simulink model "simulation_diego_perea"  (R2020a)
settings: Solver=VariableStepAuto  StartTime=0.0  StopTime=5  RelTol=1e-3
values from neighbouring files (symbols this model uses):
  a = eval(aj)    [Proyecto_diego_perea_control2.m]
  b = [1/10;0;0]    [Proyecto_diego_perea_control2.m]
  c = [0,0,1]    [Proyecto_diego_perea_control2.m]
  d = 0    [Proyecto_diego_perea_control2.m]
  h = h'    [Proyecto_diego_perea_control2.m]
  hdis = hdis'    [Proyecto_diego_perea_control2.m]
  k = place(a,b,pd)    [Proyecto_diego_perea_control2.m]
  kdis = place(adis,bdis,polosdiscredes)    [Proyecto_diego_perea_control2.m]
  ki = kt(1:1,4:4)    [Proyecto_diego_perea_control2.m]
  kidis = ktdis(:,4:4)    [Proyecto_diego_perea_control2.m]
  kp = kt(1:1,1:3)    [Proyecto_diego_perea_control2.m]
  kpdis = ktdis(:,1:3)    [Proyecto_diego_perea_control2.m]
  tm = 0.1    [Proyecto_diego_perea_control2.m]
undefined symbols (not defined in the file or in its folder): adis, bdis, cdis
settings Model: Creator=estra  LastModifiedBy=User

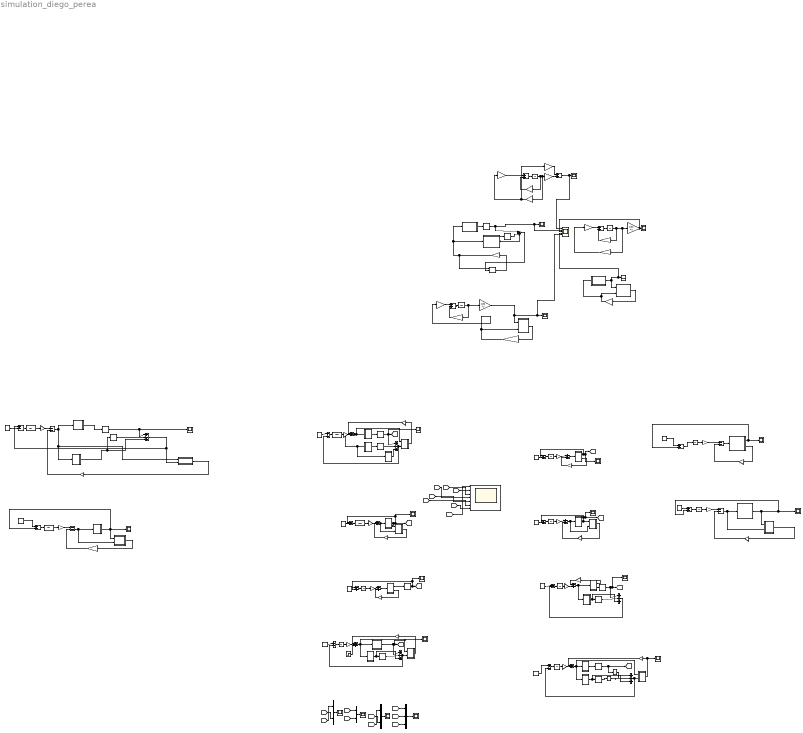
== system simulation_diego_perea ==
  note: TRACKERS (DISCRETE , CONTINUOS -SMITH)
  note: DIEGO IVAN PEREA MONTEALEGRE
  note: Continuous plant Regulator
  note: Continuous plant with regulator discrete
  note: REGULATORS
  note: Continuous plant regulator with observer
  note: Regulator with continuous plant ,observe and predictor smith.
  note: Discrete regulator with non_linear plant and with observer in discrete
  note: Tracker in discrete with linear plant and with observer in discrete
  note: Tracker with linear plant
  note: Tracker with linear plant and observer
  note: Tracker in discrete with linear plant in discrete with observer in discrete
  note: Tracker with linear plant and observer
  note: Tracker with linear plant
  note: Tracker in discrete with linear plant in discrete with observer in discrete
  note: Tracker in discrete with linear plant and with observer in discrete
  note: Plant with retard
  note: Tracker with retard smith
  note: Tracker observer smith
  note: Tracker observer smith with external perturbation
  -kp{,1,4..5,7,9} (6 alike) : Gain  Gain=-kp  Multiplication=Matrix(K*u) (u vector)
  -kp3 : Gain  Gain=-kpdis  Multiplication=Matrix(K*u) (u vector)  SampleTime=tm
  -kp6 : Gain  Gain=-kpdis  Multiplication=Matrix(K*u) (u vector)  SampleTime=tm
  Add : Sum
  Add{1,8,24,44} (4 alike) : Sum  Inputs=+-
  Add14 : Sum
  Add{6,9,25,45} (4 alike) : Sum  Inputs=--
  Add7 : Sum
  Constant{,1,3..4,6..7,9..11,21} (10 alike) : Constant
  Constant5 : Constant  SampleTime=tm
  Constant8 : Constant  SampleTime=tm
  "Continuous plant Regulator " : Sum
  Continuous plant regulator with observer : Subsystem
  "Continuous plant with regulator  discrete " : Gain  Gain=cdis  Multiplication=Matrix(K*u) (u vector)
  Discrete Transfer Fcn1 : DiscreteTransferFcn  Numerator=[1 0]  Denominator=[1 -1]  SampleTime=tm
  Discrete Transfer Fcn10 : DiscreteTransferFcn  Numerator=[1,0]  Denominator=[1 -1]  SampleTime=tm
  Discrete Transfer Fcn3 : DiscreteTransferFcn  Numerator=[1 0]  Denominator=[1 -1]  SampleTime=tm
  Discrete Transfer Fcn6 : DiscreteTransferFcn  Numerator=[1,0]  Denominator=[1 -1]  SampleTime=tm
  Discrete regulator with non_linear plant and with observer in discrete : Gain  Gain=cdis  Multiplication=Matrix(K*u) (u vector)
  Gain{,1,5..6,8,10} (6 alike) : Gain  Gain=-ki  Multiplication=Matrix(K*u) (u vector)
  Gain4 : Gain  Gain=-kidis  Multiplication=Matrix(K*u) (u vector)  SampleTime=tm
  Gain7 : Gain  Gain=-kidis  Multiplication=Matrix(K*u) (u vector)  SampleTime=tm
  Integrator : Integrator  InitialCondition=5
  Integrator{1..8} (8 alike) : Integrator
  Mux : Mux  Inputs=2
  Mux1 : Mux  Inputs=2
  Mux2 : Mux  Inputs=2
  Mux3 : Mux  Inputs=3
  Ob_predictor_smith_regulator : Subsystem
  Observer_1 : Subsystem
  Plant  with retard : TransportDelay
  Planta lineal continua12 : Subsystem
  Planta lineal continua2 : Subsystem
  Planta lineal continua3 : Subsystem
  Planta lineal continua4 : Subsystem
  Planta lineal continua7 : Subsystem
  Planta lineal continua8 : Subsystem
  Planta lineal discreta3 : Subsystem
  Planta lineal discreta4 : Subsystem
  Planta lineal discreta5 : Subsystem
  Regulator_continuos_observe_preditor smith : TransportDelay
  Retardo de la planta{1,3,5,7} (4 alike) : TransportDelay
  Scope : Scope  NumInputPorts=7
  Scope{1..10,12..22} (21 alike) : Scope
  Scope11 : Scope  NumInputPorts=5
  Step : Step  Time=0  After=0  SampleTime=0
  Sum{,7,15..16,21,26} (6 alike) : Sum  Inputs=|+-+
  Sum{1,3,8,17} (4 alike) : Sum  Inputs=|-+
  Sum{10,12,14,24} (4 alike) : Sum  Inputs=|+-
  Sum{2,4,9,11,13,18..19} (7 alike) : Sum  Inputs=|++
  Sum25 : Sum  Inputs=|+++
  Tracker  observer smith with external  perturbation : Subsystem
  Tracker  with retard smith : TransportDelay
  Tracker in discrete with linear plant and with observer in discrete : TransportDelay
  Tracker in discrete with linear plant and with observer in discrete1 : TransportDelay  DelayTime=0.8
  Tracker in discrete with linear plant in discrete with observer in discrete : Subsystem
  Tracker in discrete with linear plant in discrete with observer in discrete1 : Subsystem
  Tracker observer smith : TransportDelay
  Tracker with linear plant : Subsystem
  Tracker with linear plant and observer : Subsystem
  Tracker with linear plant and observer1 : Subsystem
  Tracker with linear plant1 : Subsystem
  Transfer Fcn : TransferFcn  Denominator=[50 1]
  Transfer Fcn1 : TransferFcn  Denominator=[50,1]
  Transport Delay1 : TransportDelay
  Transport Delay15 : TransportDelay  DelayTime=0.8
  Unit Delay : UnitDelay  InitialCondition=-8  SampleTime=tm  HasFrameUpgradeWarning=on
  Unit Delay1 : UnitDelay  InitialCondition=-8  SampleTime=tm  HasFrameUpgradeWarning=on
  a : Gain  Gain=a  Multiplication=Matrix(K*u) (u vector)
  adis : Gain  Gain=adis  Multiplication=Matrix(K*u) (u vector)
  adis1 : Gain  Gain=adis  Multiplication=Matrix(K*u) (u vector)
  b : Gain  Gain=b  Multiplication=Matrix(K*u) (u vector)
  bdis : Gain  Gain=bdis  Multiplication=Matrix(K*u) (u vector)
  bdis1 : Gain  Gain=bdis  Multiplication=Matrix(K*u) (u vector)
  c : Gain  Gain=c  Multiplication=Matrix(K*u) (u vector)
  continuous plant 6 : Subsystem
  continuous plant _ j : Subsystem
  d : Gain  Gain=d  Multiplication=Matrix(K*u) (u vector)
  k : Gain  Gain=-k  Multiplication=Matrix(K*u) (u vector)
  k3 : Gain  Gain=-k  Multiplication=Matrix(K*u) (u vector)
  k6 : Gain  Gain=-kdis  Multiplication=Matrix(K*u) (u vector)
  k8 : Gain  Gain=-k  Multiplication=Matrix(K*u) (u vector)
  kdis : Gain  Gain=-kdis  Multiplication=Matrix(K*u) (u vector)
  ki2 : Gain  Gain=ki  Multiplication=Matrix(K*u) (u vector)
  ki3 : Gain  Gain=ki  Multiplication=Matrix(K*u) (u vector)
  kidis10 : Gain  Gain=kidis  Multiplication=Matrix(K*u) (u vector)
  kidis6 : Gain  Gain=kidis  Multiplication=Matrix(K*u) (u vector)
  kp3 : Gain  Gain=kp  Multiplication=Matrix(K*u) (u vector)
  kp4 : Gain  Gain=kp  Multiplication=Matrix(K*u) (u vector)
  kpdis3 : Gain  Gain=kpdis  Multiplication=Matrix(K*u) (u vector)
  kpdis7 : Gain  Gain=kpdis  Multiplication=Matrix(K*u) (u vector)
  ob_discr_11 : Subsystem
  observador1 : Subsystem
  observador2 : Subsystem
  observador3 : Subsystem
  observadordis : Subsystem
  observadordis2 : Subsystem
  observer10 : Subsystem
  observer18 : Subsystem
  observer3 : Subsystem
  plant_1 : Subsystem
  planta13 : Subsystem
  wires:
  Continuous plant regulator with observer/1(Out1) -> Scope11/4, Scope10/1, Observer_1/1(In2)
  k3/1 -> Continuous plant regulator with observer/1(In1), Observer_1/2(In1)
  Observer_1/1(Out1) -> k3/1
  Transport Delay1/1 -> Sum/2
  plant_1/1(Out1) -> Transport Delay1/1, Sum/3
  k8/1 -> continuous plant _ j/1(In1), plant_1/1(In1), Ob_predictor_smith_regulator/1(In1)
  Ob_predictor_smith_regulator/1(Out1) -> k8/1
  Regulator_continuos_observe_preditor smith/1 -> Scope11/2, Scope8/1, Sum/1
  continuous plant _ j/1(Out1) -> Regulator_continuos_observe_preditor smith/1
  Sum/1 -> Ob_predictor_smith_regulator/2(In2)
  c/1 -> "Continuous plant Regulator "/2
  Add/1 -> Integrator/1
  b/1 -> Add/1
  a/1 -> Add/2
  k/1 -> d/1, b/1
  d/1 -> "Continuous plant Regulator "/1
  Integrator/1 -> a/1, k/1, c/1
  kdis/1 -> bdis/1
  adis/1 -> Add14/2
  Add14/1 -> Unit Delay/1
  Unit Delay/1 -> kdis/1, "Continuous plant with regulator  discrete "/1, adis/1
  bdis/1 -> Add14/1
  k6/1 -> bdis1/1, ob_discr_11/2(In1)
  ob_discr_11/1(Out1) -> k6/1
  continuous plant 6/1(Out1) -> Tracker in discrete with linear plant and with observer in discrete1/1
  Constant21/1 -> Add44/1
  Sum7/1 -> observer18/2(In2), Add44/2
  kidis10/1 -> Add45/1
  observer18/1(Out1) -> kpdis7/1
  Tracker in discrete with linear plant and with observer in discrete1/1 -> Scope3/1, Sum7/1
  Add44/1 -> Discrete Transfer Fcn10/1
  Discrete Transfer Fcn10/1 -> kidis10/1
  Add45/1 -> planta13/1(In1), observer18/1(In1), continuous plant 6/1(In1)
  kpdis7/1 -> Add45/2
  Transport Delay15/1 -> Sum7/2
  planta13/1(Out1) -> Sum7/3, Transport Delay15/1
  Add6/1 -> Tracker with linear plant1/1(In1)
  kp4/1 -> Add6/2
  Tracker with linear plant1/2(Output) -> kp4/1
  Integrator1/1 -> ki3/1
  Add1/1 -> Integrator1/1
  ki3/1 -> Add6/1
  Constant3/1 -> Add1/1
  Add9/1 -> observer3/2(In1), Tracker with linear plant and observer1/1(In1)
  kp3/1 -> Add9/2
  Constant4/1 -> Add8/1
  observer3/1(Out1) -> kp3/1
  Integrator7/1 -> ki2/1
  Add8/1 -> Integrator7/1
  ki2/1 -> Add9/1
  Tracker with linear plant and observer1/1(Out1) -> Scope12/1, Add8/2, observer3/1(In2)
  Tracker in discrete with linear plant in discrete with observer in discrete1/1(Out1) -> Scope4/1, observer10/1(In2), Add24/2
  kpdis3/1 -> Add25/2
  Add25/1 -> observer10/2(In1), Tracker in discrete with linear plant in discrete with observer in discrete1/1(In1)
  observer10/1(Out1) -> kpdis3/1
  Discrete Transfer Fcn6/1 -> kidis6/1
  Constant11/1 -> Add24/1
  kidis6/1 -> Add25/1
  Add24/1 -> Discrete Transfer Fcn6/1
  Discrete regulator with non_linear plant and with observer in discrete/1 -> Scope11/5, Scope9/1, ob_discr_11/1(In2)
  Tracker with linear plant1/1(Out1) -> Scope14/1, Add1/2
  Add7/1 -> Unit Delay1/1
  adis1/1 -> Add7/2
  Unit Delay1/1 -> Discrete regulator with non_linear plant and with observer in discrete/1, adis1/1
  bdis1/1 -> Add7/1
  "Continuous plant with regulator  discrete "/1 -> Scope11/3, Scope7/1
  "Continuous plant Regulator "/1 -> Scope11/1, Scope6/1
  Discrete Transfer Fcn3/1 -> Gain7/1
  Retardo de la planta7/1 -> Sum26/2
  -kp1/1 -> Sum4/2
  Planta lineal continua12/1(y) -> Sum26/3, Retardo de la planta7/1
  Sum25/1 -> Tracker  observer smith with external  perturbation/1(In1), observador3/1(u), Planta lineal continua12/1(u)
  Constant10/1 -> Sum24/1
  Constant8/1 -> Sum12/1
  Retardo de la planta1/1 -> Sum15/2
  Sum19/1 -> Planta lineal continua8/1(u), Planta lineal continua7/1(u)
  Planta lineal discreta5/1(y) -> Sum15/3
  Planta lineal continua8/1(y) -> Sum21/3, Retardo de la planta3/1
  Integrator4/1 -> Gain5/1
  Constant9/1 -> Sum14/1
  Tracker with linear plant/2(x) -> -kp/1
  Sum14/1 -> Integrator6/1
  Sum9/1 -> Tracker in discrete with linear plant in discrete with observer in discrete/1(u), observadordis/2(u)
  Gain4/1 -> Sum9/1
  Gain5/1 -> Sum18/1
  Sum18/1 -> Planta lineal continua2/1(u)
  Gain1/1 -> Sum4/1
  Sum8/1 -> Discrete Transfer Fcn1/1
  Integrator2/1 -> Gain/1
  Tracker  with retard smith/1 -> Sum21/1, Scope17/1, [A2]
  Integrator6/1 -> Gain8/1
  Planta lineal continua4/1(y) -> Sum16/3, Retardo de la planta5/1
  Planta lineal discreta4/1(y) -> Retardo de la planta1/1
  Retardo de la planta3/1 -> Sum21/2
  Sum1/1 -> Integrator2/1
  -kp4/1 -> Sum18/2
  [B1] -> Mux3/1
  -kp5/1 -> Sum11/1
  [C2] -> Mux3/2
  observadordis2/1(xgorro) -> -kp6/1
  Discrete Transfer Fcn1/1 -> Gain4/1
  -kp7/1 -> Sum19/1
  Constant5/1 -> Sum8/2
  Sum26/1 -> Sum24/2, observador3/2(y)
  [A1] -> Mux/2
  Sum11/1 -> Planta lineal continua4/1(u), Planta lineal continua3/1(u), observador2/1(u)
  Integrator3/1 -> Gain1/1
  Plant  with retard/1 -> Scope16/1, Sum17/1, [A1]
  Planta lineal continua7/1(x) -> -kp7/1
  [C1] -> Mux2/2
  -kp9/1 -> Sum25/1
  Sum12/1 -> Discrete Transfer Fcn3/1
  Gain10/1 -> Sum25/2
  [B1] -> Mux1/2
  Mux1/1 -> Scope13/1
  Sum24/1 -> Integrator8/1
  Mux/1 -> Scope5/1
  observador1/1(xgorro) -> -kp1/1
  Planta lineal discreta3/1(y) -> Tracker in discrete with linear plant and with observer in discrete/1
  Integrator8/1 -> Gain10/1
  Planta lineal continua2/1(y) -> Plant  with retard/1
  Sum15/1 -> Sum12/2, observadordis2/2(y)
  Sum3/1 -> Integrator3/1
  Integrator5/1 -> Gain6/1
  -kp3/1 -> Sum9/2
  Sum10/1 -> Integrator5/1
  Gain7/1 -> Sum13/2
  Planta lineal continua2/2(x) -> -kp4/1
  -kp/1 -> Sum2/2
  Tracker observer smith/1 -> Transfer Fcn1/1, [F]
  Tracker in discrete with linear plant and with observer in discrete/1 -> Scope21/1, Sum15/1, [C2]
  Retardo de la planta5/1 -> Transfer Fcn/1
  observadordis/1(xgorro) -> -kp3/1
  Constant1/1 -> Sum3/2
  Sum4/1 -> Tracker with linear plant and observer/1(u), observador1/2(u)
  Constant7/1 -> Sum10/1
  Mux3/1 -> Scope2/1
  [F] -> Mux3/3
  Step/1 -> Sum25/3
  Sum13/1 -> Planta lineal discreta3/1(u), observadordis2/1(u), Planta lineal discreta5/1(u), Planta lineal discreta4/1(u)
  observador3/1(xgorro) -> -kp9/1
  Tracker with linear plant/1(y) -> Sum1/1, [D], Scope15/1
  -kp6/1 -> Sum13/1
  Gain6/1 -> Sum11/2
  observador2/1(xgorro) -> Scope20/1, -kp5/1
  Sum17/1 -> Integrator4/1
  Sum16/1 -> observador2/2(y), Sum10/2
  Transfer Fcn1/1 -> Sum16/1
  Sum21/1 -> Sum14/2
  Gain8/1 -> Sum19/2
  Transfer Fcn/1 -> Sum16/2
  Constant/1 -> Sum1/2
  Constant6/1 -> Sum17/2
  Mux2/1 -> Scope1/1
  Tracker  observer smith with external  perturbation/1(Out1) -> Scope18/1, [B1], Sum26/1
  Sum2/1 -> Tracker with linear plant/1(u)
  [B] -> Mux1/1
  Planta lineal continua7/2(y) -> Tracker  with retard smith/1
  Planta lineal continua3/1(y) -> Tracker observer smith/1
  Gain/1 -> Sum2/1
  [A2] -> Mux/1
  [C2] -> Mux2/1
  Tracker in discrete with linear plant in discrete with observer in discrete/1(y) -> Scope19/1, Sum8/1, [C1], observadordis/1(y)
  Tracker with linear plant and observer/1(y) -> Scope22/1, [B], Sum3/1, observador1/1(y)
  [A2] -> Scope/2
  [B] -> Scope/3
  [B1] -> Scope/4
  [C1] -> Scope/5
  [C2] -> Scope/6
  [F] -> Scope/7
  [D] -> Scope/1

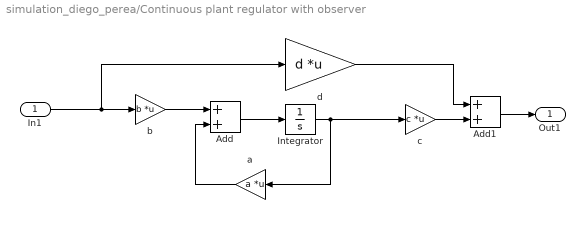
== system simulation_diego_perea/Continuous plant regulator with observer ==
  In1 : Inport
  Add : Sum
  Add1 : Sum
  Integrator : Integrator  InitialCondition=20
  a : Gain  Gain=a  Multiplication=Matrix(K*u) (u vector)
  b : Gain  Gain=b  Multiplication=Matrix(K*u) (u vector)
  c : Gain  Gain=c  Multiplication=Matrix(K*u) (u vector)
  d : Gain  Gain=d  Multiplication=Matrix(K*u) (u vector)
  Out1 : Outport
  wires:
  Integrator/1 -> c/1, a/1
  a/1 -> Add/2
  b/1 -> Add/1
  Add/1 -> Integrator/1
  In1/1 -> d/1, b/1
  c/1 -> Add1/2
  d/1 -> Add1/1
  Add1/1 -> Out1/1

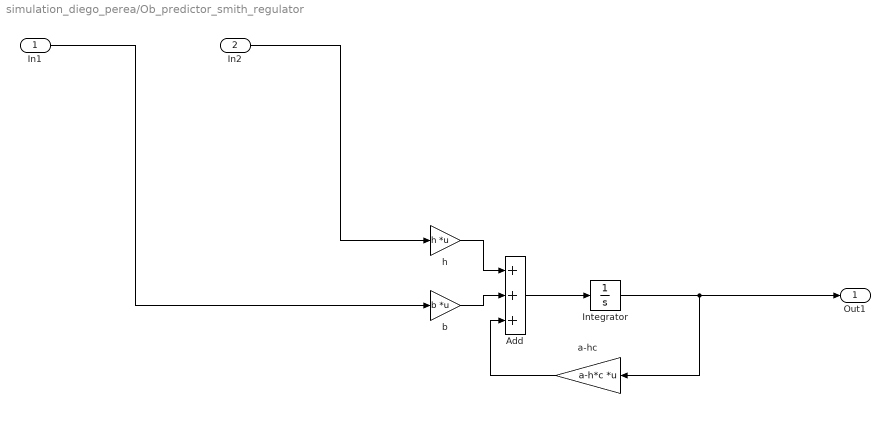
== system simulation_diego_perea/Ob_predictor_smith_regulator ==
  In1 : Inport
  In2 : Inport  Port=2
  Add : Sum  Inputs=+++
  Integrator : Integrator  InitialCondition=4
  a-hc : Gain  Gain=a-h*c  Multiplication=Matrix(K*u) (u vector)
  b : Gain  Gain=b  Multiplication=Matrix(K*u) (u vector)
  h : Gain  Gain=h  Multiplication=Matrix(K*u) (u vector)
  Out1 : Outport
  wires:
  a-hc/1 -> Add/3
  b/1 -> Add/2
  In2/1 -> h/1
  Integrator/1 -> Out1/1, a-hc/1
  In1/1 -> b/1
  Add/1 -> Integrator/1
  h/1 -> Add/1

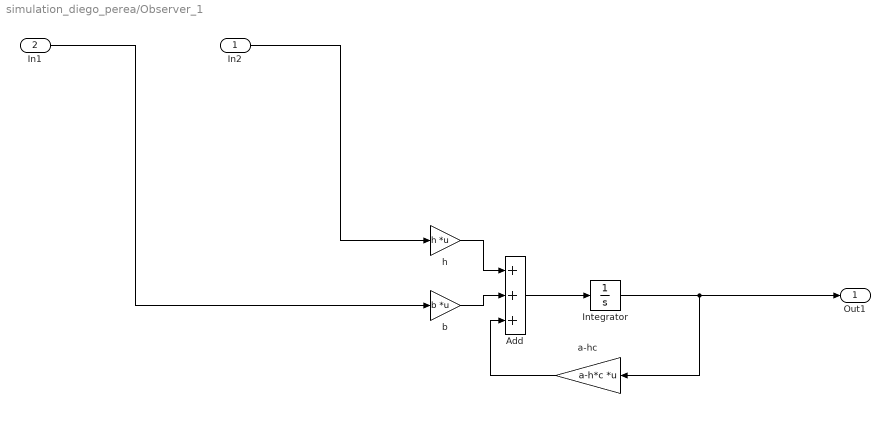
== system simulation_diego_perea/Observer_1 ==
  In2 : Inport
  In1 : Inport  Port=2
  Add : Sum  Inputs=+++
  Integrator : Integrator  InitialCondition=8
  a-hc : Gain  Gain=a-h*c  Multiplication=Matrix(K*u) (u vector)
  b : Gain  Gain=b  Multiplication=Matrix(K*u) (u vector)
  h : Gain  Gain=h  Multiplication=Matrix(K*u) (u vector)
  Out1 : Outport
  wires:
  a-hc/1 -> Add/3
  b/1 -> Add/2
  In2/1 -> h/1
  Integrator/1 -> Out1/1, a-hc/1
  In1/1 -> b/1
  Add/1 -> Integrator/1
  h/1 -> Add/1

== system simulation_diego_perea/Planta lineal continua12 ==
  u : Inport
  A : Gain  Gain=a  Multiplication=Matrix(K*u) (u vector)
  B : Gain  Gain=b  Multiplication=Matrix(K*u) (u vector)
  C : Gain  Gain=c  Multiplication=Matrix(K*u) (u vector)
  Integrator : Integrator
  Sum : Sum  Inputs=|++
  y : Outport
  wires:
  C/1 -> y/1
  u/1 -> B/1
  Integrator/1 -> C/1, A/1
  A/1 -> Sum/2
  Sum/1 -> Integrator/1
  B/1 -> Sum/1

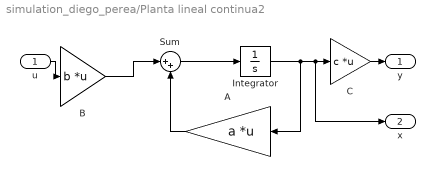
== system simulation_diego_perea/Planta lineal continua2 ==
  u : Inport
  A : Gain  Gain=a  Multiplication=Matrix(K*u) (u vector)
  B : Gain  Gain=b  Multiplication=Matrix(K*u) (u vector)
  C : Gain  Gain=c  Multiplication=Matrix(K*u) (u vector)
  Integrator : Integrator
  Sum : Sum  Inputs=|++
  y : Outport
  x : Outport  Port=2
  wires:
  C/1 -> y/1
  u/1 -> B/1
  Integrator/1 -> x/1, C/1, A/1
  A/1 -> Sum/2
  Sum/1 -> Integrator/1
  B/1 -> Sum/1

== system simulation_diego_perea/Planta lineal continua3 ==
  u : Inport
  A : Gain  Gain=a  Multiplication=Matrix(K*u) (u vector)
  B : Gain  Gain=b  Multiplication=Matrix(K*u) (u vector)
  C : Gain  Gain=c  Multiplication=Matrix(K*u) (u vector)
  Integrator : Integrator
  Sum : Sum  Inputs=|++
  y : Outport
  wires:
  B/1 -> Sum/1
  Sum/1 -> Integrator/1
  A/1 -> Sum/2
  Integrator/1 -> C/1, A/1
  u/1 -> B/1
  C/1 -> y/1

== system simulation_diego_perea/Planta lineal continua4 ==
  u : Inport
  A : Gain  Gain=a  Multiplication=Matrix(K*u) (u vector)
  B : Gain  Gain=b  Multiplication=Matrix(K*u) (u vector)
  C : Gain  Gain=c  Multiplication=Matrix(K*u) (u vector)
  Integrator : Integrator
  Sum : Sum  Inputs=|++
  y : Outport
  wires:
  B/1 -> Sum/1
  Sum/1 -> Integrator/1
  A/1 -> Sum/2
  Integrator/1 -> A/1, C/1
  u/1 -> B/1
  C/1 -> y/1

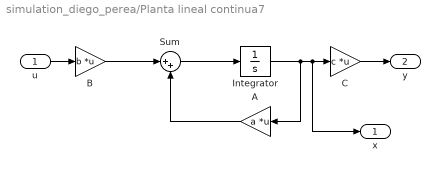
== system simulation_diego_perea/Planta lineal continua7 ==
  u : Inport
  A : Gain  Gain=a  Multiplication=Matrix(K*u) (u vector)
  B : Gain  Gain=b  Multiplication=Matrix(K*u) (u vector)
  C : Gain  Gain=c  Multiplication=Matrix(K*u) (u vector)
  Integrator : Integrator
  Sum : Sum  Inputs=|++
  x : Outport
  y : Outport  Port=2
  wires:
  u/1 -> B/1
  Integrator/1 -> x/1, C/1, A/1
  A/1 -> Sum/2
  Sum/1 -> Integrator/1
  B/1 -> Sum/1
  C/1 -> y/1

== system simulation_diego_perea/Planta lineal continua8 ==
  u : Inport
  A : Gain  Gain=a  Multiplication=Matrix(K*u) (u vector)
  B : Gain  Gain=b  Multiplication=Matrix(K*u) (u vector)
  C : Gain  Gain=c  Multiplication=Matrix(K*u) (u vector)
  Integrator : Integrator
  Sum : Sum  Inputs=|++
  y : Outport
  wires:
  B/1 -> Sum/1
  Sum/1 -> Integrator/1
  A/1 -> Sum/2
  Integrator/1 -> A/1, C/1
  u/1 -> B/1
  C/1 -> y/1

== system simulation_diego_perea/Planta lineal discreta3 ==
  u : Inport
  Sum4 : Sum  Inputs=|++
  Unit Delay : UnitDelay  SampleTime=-1  HasFrameUpgradeWarning=on
  adis : Gain  Gain=adis  Multiplication=Matrix(K*u) (u vector)  SampleTime=tm
  bdis : Gain  Gain=bdis  Multiplication=Matrix(K*u) (u vector)  SampleTime=tm
  cdis : Gain  Gain=cdis  Multiplication=Matrix(K*u) (u vector)  SampleTime=tm
  y : Outport
  wires:
  cdis/1 -> y/1
  u/1 -> bdis/1
  adis/1 -> Sum4/2
  Unit Delay/1 -> cdis/1, adis/1
  Sum4/1 -> Unit Delay/1
  bdis/1 -> Sum4/1

== system simulation_diego_perea/Planta lineal discreta4 ==
  u : Inport
  Sum4 : Sum  Inputs=|++
  Unit Delay : UnitDelay  SampleTime=-1  HasFrameUpgradeWarning=on
  adis : Gain  Gain=adis  Multiplication=Matrix(K*u) (u vector)  SampleTime=tm
  bdis : Gain  Gain=bdis  Multiplication=Matrix(K*u) (u vector)  SampleTime=tm
  cdis : Gain  Gain=cdis  Multiplication=Matrix(K*u) (u vector)  SampleTime=tm
  y : Outport
  wires:
  cdis/1 -> y/1
  u/1 -> bdis/1
  adis/1 -> Sum4/2
  Unit Delay/1 -> cdis/1, adis/1
  Sum4/1 -> Unit Delay/1
  bdis/1 -> Sum4/1

== system simulation_diego_perea/Planta lineal discreta5 ==
  u : Inport
  Sum4 : Sum  Inputs=|++
  Unit Delay : UnitDelay  SampleTime=-1  HasFrameUpgradeWarning=on
  adis : Gain  Gain=adis  Multiplication=Matrix(K*u) (u vector)  SampleTime=tm
  bdis : Gain  Gain=bdis  Multiplication=Matrix(K*u) (u vector)  SampleTime=tm
  cdis : Gain  Gain=cdis  Multiplication=Matrix(K*u) (u vector)  SampleTime=tm
  y : Outport
  wires:
  bdis/1 -> Sum4/1
  Sum4/1 -> Unit Delay/1
  Unit Delay/1 -> adis/1, cdis/1
  adis/1 -> Sum4/2
  u/1 -> bdis/1
  cdis/1 -> y/1

== system simulation_diego_perea/Tracker  observer smith with external  perturbation ==
  In1 : Inport
  Planta lineal continua11 : Subsystem
  Retardo de la planta8 : TransportDelay
  Out1 : Outport
  wires:
  Retardo de la planta8/1 -> Out1/1
  In1/1 -> Planta lineal continua11/1(u)
  Planta lineal continua11/1(y) -> Retardo de la planta8/1

== system simulation_diego_perea/Tracker in discrete with linear plant in discrete with observer in discrete ==
  u : Inport
  Sum4 : Sum  Inputs=|++
  Unit Delay : UnitDelay  SampleTime=-1  HasFrameUpgradeWarning=on
  adis : Gain  Gain=adis  Multiplication=Matrix(K*u) (u vector)  SampleTime=tm
  bdis : Gain  Gain=bdis  Multiplication=Matrix(K*u) (u vector)  SampleTime=tm
  cdis : Gain  Gain=cdis  Multiplication=Matrix(K*u) (u vector)  SampleTime=tm
  y : Outport
  wires:
  cdis/1 -> y/1
  u/1 -> bdis/1
  adis/1 -> Sum4/2
  Unit Delay/1 -> cdis/1, adis/1
  Sum4/1 -> Unit Delay/1
  bdis/1 -> Sum4/1

== system simulation_diego_perea/Tracker in discrete with linear plant in discrete with observer in discrete1 ==
  In1 : Inport
  Add14 : Sum
  Unit Delay : UnitDelay  SampleTime=tm  HasFrameUpgradeWarning=on
  adis : Gain  Gain=adis  Multiplication=Matrix(K*u) (u vector)
  bdis : Gain  Gain=bdis  Multiplication=Matrix(K*u) (u vector)
  cdis : Gain  Gain=cdis  Multiplication=Matrix(K*u) (u vector)
  Out1 : Outport
  wires:
  adis/1 -> Add14/2
  Add14/1 -> Unit Delay/1
  bdis/1 -> Add14/1
  Unit Delay/1 -> cdis/1, adis/1
  cdis/1 -> Out1/1
  In1/1 -> bdis/1

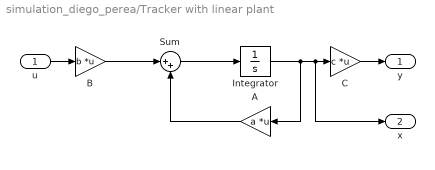
== system simulation_diego_perea/Tracker with linear plant ==
  u : Inport
  A : Gain  Gain=a  Multiplication=Matrix(K*u) (u vector)
  B : Gain  Gain=b  Multiplication=Matrix(K*u) (u vector)
  C : Gain  Gain=c  Multiplication=Matrix(K*u) (u vector)
  Integrator : Integrator
  Sum : Sum  Inputs=|++
  y : Outport
  x : Outport  Port=2
  wires:
  B/1 -> Sum/1
  Sum/1 -> Integrator/1
  A/1 -> Sum/2
  Integrator/1 -> A/1, C/1, x/1
  u/1 -> B/1
  C/1 -> y/1

== system simulation_diego_perea/Tracker with linear plant and observer ==
  u : Inport
  A : Gain  Gain=a  Multiplication=Matrix(K*u) (u vector)
  B : Gain  Gain=b  Multiplication=Matrix(K*u) (u vector)
  C : Gain  Gain=c  Multiplication=Matrix(K*u) (u vector)
  Integrator : Integrator
  Sum : Sum  Inputs=|++
  y : Outport
  wires:
  C/1 -> y/1
  u/1 -> B/1
  Integrator/1 -> A/1, C/1
  A/1 -> Sum/2
  Sum/1 -> Integrator/1
  B/1 -> Sum/1

== system simulation_diego_perea/Tracker with linear plant and observer1 ==
  In1 : Inport
  Add : Sum
  Integrator : Integrator
  a : Gain  Gain=a  Multiplication=Matrix(K*u) (u vector)
  b : Gain  Gain=b  Multiplication=Matrix(K*u) (u vector)
  c : Gain  Gain=c  Multiplication=Matrix(K*u) (u vector)
  Out1 : Outport
  wires:
  c/1 -> Out1/1
  Integrator/1 -> c/1, a/1
  a/1 -> Add/2
  b/1 -> Add/1
  Add/1 -> Integrator/1
  In1/1 -> b/1

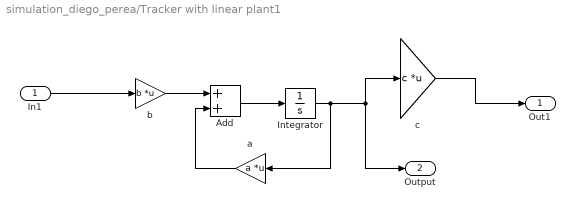
== system simulation_diego_perea/Tracker with linear plant1 ==
  In1 : Inport
  Add : Sum
  Integrator : Integrator
  a : Gain  Gain=a  Multiplication=Matrix(K*u) (u vector)
  b : Gain  Gain=b  Multiplication=Matrix(K*u) (u vector)
  c : Gain  Gain=c  Multiplication=Matrix(K*u) (u vector)
  Out1 : Outport
  Output : Outport  Port=2  VectorParamsAs1DForOutWhenUnconnected=off
  wires:
  c/1 -> Out1/1
  Integrator/1 -> Output/1, c/1, a/1
  a/1 -> Add/2
  b/1 -> Add/1
  Add/1 -> Integrator/1
  In1/1 -> b/1

== system simulation_diego_perea/continuous plant 6 ==
  In1 : Inport
  Add : Sum
  Unit Delay : UnitDelay  SampleTime=tm  HasFrameUpgradeWarning=on
  adis : Gain  Gain=adis  Multiplication=Matrix(K*u) (u vector)
  bdis : Gain  Gain=bdis  Multiplication=Matrix(K*u) (u vector)
  cdis : Gain  Gain=cdis  Multiplication=Matrix(K*u) (u vector)
  Out1 : Outport
  wires:
  In1/1 -> bdis/1
  Add/1 -> Unit Delay/1
  bdis/1 -> Add/1
  adis/1 -> Add/2
  Unit Delay/1 -> cdis/1, adis/1
  cdis/1 -> Out1/1

== system simulation_diego_perea/continuous plant _ j ==
  In1 : Inport
  Add : Sum
  Integrator : Integrator  InitialCondition=9
  a : Gain  Gain=a  Multiplication=Matrix(K*u) (u vector)
  b : Gain  Gain=b  Multiplication=Matrix(K*u) (u vector)
  c : Gain  Gain=c  Multiplication=Matrix(K*u) (u vector)
  Out1 : Outport
  wires:
  c/1 -> Out1/1
  Integrator/1 -> c/1, a/1
  a/1 -> Add/2
  b/1 -> Add/1
  Add/1 -> Integrator/1
  In1/1 -> b/1

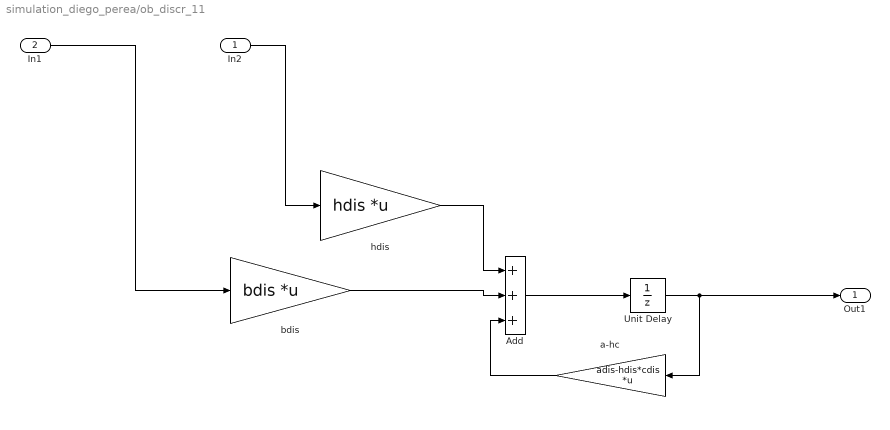
== system simulation_diego_perea/ob_discr_11 ==
  In2 : Inport
  In1 : Inport  Port=2
  Add : Sum  Inputs=+++
  Unit Delay : UnitDelay  InitialCondition=2  SampleTime=tm  HasFrameUpgradeWarning=on
  a-hc : Gain  Gain=adis-hdis*cdis  Multiplication=Matrix(K*u) (u vector)
  bdis : Gain  Gain=bdis  Multiplication=Matrix(K*u) (u vector)
  hdis : Gain  Gain=hdis  Multiplication=Matrix(K*u) (u vector)
  Out1 : Outport
  wires:
  a-hc/1 -> Add/3
  bdis/1 -> Add/2
  In2/1 -> hdis/1
  Unit Delay/1 -> Out1/1, a-hc/1
  In1/1 -> bdis/1
  Add/1 -> Unit Delay/1
  hdis/1 -> Add/1

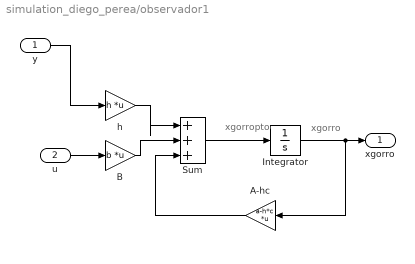
== system simulation_diego_perea/observador1 ==
  note: xgorro
  note: xgorropto
  y : Inport
  u : Inport  Port=2
  A-hc : Gain  Gain=a-h*c  Multiplication=Matrix(K*u) (u vector)
  B : Gain  Gain=b  Multiplication=Matrix(K*u) (u vector)
  Integrator : Integrator
  Sum : Sum  Inputs=|+++
  h : Gain  Gain=h  Multiplication=Matrix(K*u) (u vector)
  xgorro : Outport
  wires:
  u/1 -> B/1
  h/1 -> Sum/1
  B/1 -> Sum/2
  A-hc/1 -> Sum/3
  Integrator/1 -> xgorro/1, A-hc/1
  Sum/1 -> Integrator/1
  y/1 -> h/1

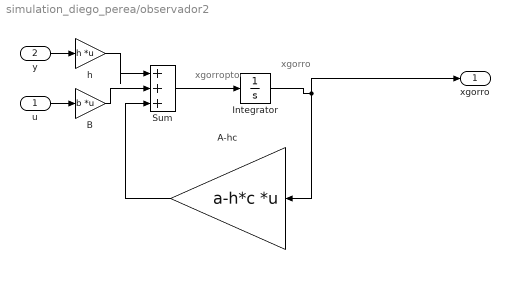
== system simulation_diego_perea/observador2 ==
  note: xgorropto
  note: xgorro
  u : Inport
  y : Inport  Port=2
  A-hc : Gain  Gain=a-h*c  Multiplication=Matrix(K*u) (u vector)
  B : Gain  Gain=b  Multiplication=Matrix(K*u) (u vector)
  Integrator : Integrator
  Sum : Sum  Inputs=|+++
  h : Gain  Gain=h  Multiplication=Matrix(K*u) (u vector)
  xgorro : Outport
  wires:
  u/1 -> B/1
  y/1 -> h/1
  Integrator/1 -> A-hc/1, xgorro/1
  Sum/1 -> Integrator/1
  A-hc/1 -> Sum/3
  B/1 -> Sum/2
  h/1 -> Sum/1

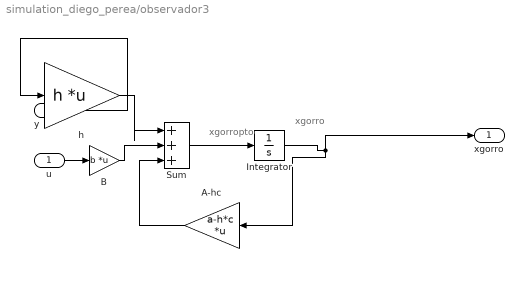
== system simulation_diego_perea/observador3 ==
  note: xgorro
  note: xgorropto
  u : Inport
  y : Inport  Port=2
  A-hc : Gain  Gain=a-h*c  Multiplication=Matrix(K*u) (u vector)
  B : Gain  Gain=b  Multiplication=Matrix(K*u) (u vector)
  Integrator : Integrator
  Sum : Sum  Inputs=|+++
  h : Gain  Gain=h  Multiplication=Matrix(K*u) (u vector)
  xgorro : Outport
  wires:
  h/1 -> Sum/1
  B/1 -> Sum/2
  A-hc/1 -> Sum/3
  Sum/1 -> Integrator/1
  Integrator/1 -> xgorro/1, A-hc/1
  y/1 -> h/1
  u/1 -> B/1

== system simulation_diego_perea/observadordis ==
  note: xgorro
  note: y
  y : Inport
  u : Inport  Port=2
  Ad-hd*cd : Gain  Gain=adis-hdis*cdis  Multiplication=Matrix(K*u) (u vector)  SampleTime=tm
  Gain27 : Gain  Gain=bdis  Multiplication=Matrix(K*u) (u vector)  SampleTime=tm
  Sum17 : Sum  Inputs=|+++
  Unit Delay : UnitDelay  SampleTime=-1  HasFrameUpgradeWarning=on
  h1 : Gain  Gain=hdis  Multiplication=Matrix(K*u) (u vector)  SampleTime=tm
  xgorro : Outport
  wires:
  Sum17/1 -> Unit Delay/1
  h1/1 -> Sum17/1
  Unit Delay/1 -> Ad-hd*cd/1, xgorro/1
  Ad-hd*cd/1 -> Sum17/3
  Gain27/1 -> Sum17/2
  y/1 -> h1/1
  u/1 -> Gain27/1

== system simulation_diego_perea/observadordis2 ==
  note: xgorro
  u : Inport
  y : Inport  Port=2
  Ad-hd*cd : Gain  Gain=adis-hdis*cdis  Multiplication=Matrix(K*u) (u vector)  SampleTime=tm
  Gain27 : Gain  Gain=bdis  Multiplication=Matrix(K*u) (u vector)  SampleTime=tm
  Sum17 : Sum  Inputs=|+++
  Unit Delay : UnitDelay  SampleTime=-1  HasFrameUpgradeWarning=on
  h1 : Gain  Gain=hdis  Multiplication=Matrix(K*u) (u vector)  SampleTime=tm
  xgorro : Outport
  wires:
  Sum17/1 -> Unit Delay/1
  h1/1 -> Sum17/1
  Unit Delay/1 -> Ad-hd*cd/1, xgorro/1
  Ad-hd*cd/1 -> Sum17/3
  Gain27/1 -> Sum17/2
  y/1 -> h1/1
  u/1 -> Gain27/1

== system simulation_diego_perea/observer10 ==
  In2 : Inport
  In1 : Inport  Port=2
  Add : Sum  Inputs=+++
  Unit Delay : UnitDelay  SampleTime=tm  HasFrameUpgradeWarning=on
  a-hc : Gain  Gain=adis-hdis*cdis  Multiplication=Matrix(K*u) (u vector)
  bdis : Gain  Gain=bdis  Multiplication=Matrix(K*u) (u vector)
  hdis : Gain  Gain=hdis  Multiplication=Matrix(K*u) (u vector)
  Out1 : Outport
  wires:
  a-hc/1 -> Add/3
  bdis/1 -> Add/2
  In2/1 -> hdis/1
  Unit Delay/1 -> Out1/1, a-hc/1
  In1/1 -> bdis/1
  Add/1 -> Unit Delay/1
  hdis/1 -> Add/1

== system simulation_diego_perea/observer18 ==
  In1 : Inport
  In2 : Inport  Port=2
  Add : Sum  Inputs=+++
  Unit Delay : UnitDelay  SampleTime=tm  HasFrameUpgradeWarning=on
  a-hc : Gain  Gain=adis-hdis*cdis  Multiplication=Matrix(K*u) (u vector)
  bdis : Gain  Gain=bdis  Multiplication=Matrix(K*u) (u vector)
  hdis : Gain  Gain=hdis  Multiplication=Matrix(K*u) (u vector)
  Out1 : Outport
  wires:
  hdis/1 -> Add/1
  Add/1 -> Unit Delay/1
  In1/1 -> bdis/1
  Unit Delay/1 -> a-hc/1, Out1/1
  In2/1 -> hdis/1
  bdis/1 -> Add/2
  a-hc/1 -> Add/3

== system simulation_diego_perea/observer3 ==
  In2 : Inport
  In1 : Inport  Port=2
  Add : Sum  Inputs=+++
  Integrator : Integrator
  a-hc : Gain  Gain=a-h*c  Multiplication=Matrix(K*u) (u vector)
  b : Gain  Gain=b  Multiplication=Matrix(K*u) (u vector)
  h : Gain  Gain=h  Multiplication=Matrix(K*u) (u vector)
  Out1 : Outport
  wires:
  a-hc/1 -> Add/3
  b/1 -> Add/2
  In2/1 -> h/1
  Integrator/1 -> Out1/1, a-hc/1
  In1/1 -> b/1
  Add/1 -> Integrator/1
  h/1 -> Add/1

== system simulation_diego_perea/plant_1 ==
  In1 : Inport
  Add : Sum
  Integrator : Integrator  InitialCondition=9
  a : Gain  Gain=a  Multiplication=Matrix(K*u) (u vector)
  b : Gain  Gain=b  Multiplication=Matrix(K*u) (u vector)
  c : Gain  Gain=c  Multiplication=Matrix(K*u) (u vector)
  Out1 : Outport
  wires:
  c/1 -> Out1/1
  Integrator/1 -> c/1, a/1
  a/1 -> Add/2
  b/1 -> Add/1
  Add/1 -> Integrator/1
  In1/1 -> b/1

== system simulation_diego_perea/planta13 ==
  In1 : Inport
  Add : Sum
  Unit Delay : UnitDelay  SampleTime=tm  HasFrameUpgradeWarning=on
  adis : Gain  Gain=adis  Multiplication=Matrix(K*u) (u vector)
  bdis : Gain  Gain=bdis  Multiplication=Matrix(K*u) (u vector)
  cdis : Gain  Gain=cdis  Multiplication=Matrix(K*u) (u vector)
  Out1 : Outport
  wires:
  In1/1 -> bdis/1
  Add/1 -> Unit Delay/1
  bdis/1 -> Add/1
  adis/1 -> Add/2
  Unit Delay/1 -> cdis/1, adis/1
  cdis/1 -> Out1/1

== system simulation_diego_perea/Tracker  observer smith with external  perturbation/Planta lineal continua11 ==
  u : Inport
  A : Gain  Gain=a  Multiplication=Matrix(K*u) (u vector)
  B : Gain  Gain=b  Multiplication=Matrix(K*u) (u vector)
  C : Gain  Gain=c  Multiplication=Matrix(K*u) (u vector)
  Integrator : Integrator
  Sum : Sum  Inputs=|++
  y : Outport
  wires:
  C/1 -> y/1
  u/1 -> B/1
  Integrator/1 -> A/1, C/1
  A/1 -> Sum/2
  Sum/1 -> Integrator/1
  B/1 -> Sum/1
